simulink model "debut_de_qq"  (R2014a)
settings: Solver=ode45  StartTime=0.0  StopTime=10.0  RelTol=1e-3
undefined symbols (not defined in the file): K, KD, r, Ti
libraries: lib_robotRP x2
settings Model: Creator=2asri13  LastModifiedBy=2asri13

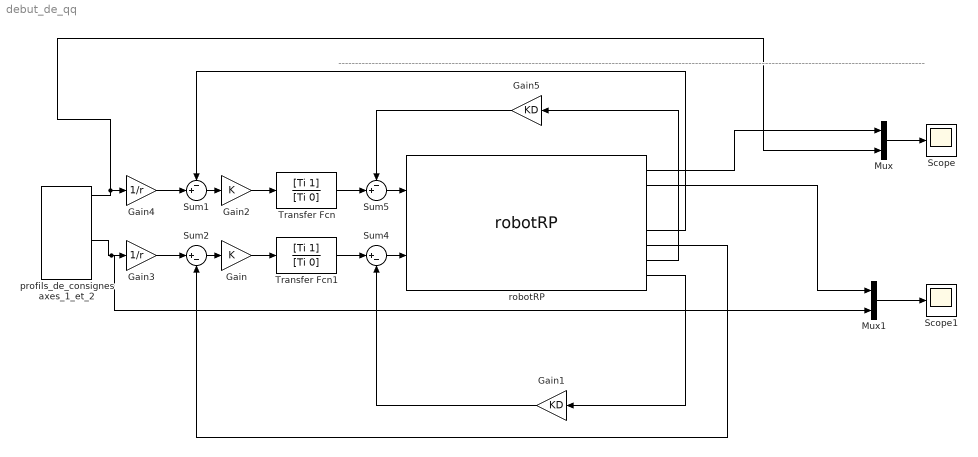
== system debut_de_qq ==
  note: --------------------------------------------------------------------------------------------------------------------------------------------------------------------------------
  Gain : Gain  Gain=K
  Gain1 : Gain  Gain=KD
  Gain2 : Gain  Gain=K
  Gain3 : Gain  Gain=1/r
  Gain4 : Gain  Gain=1/r
  Gain5 : Gain  Gain=KD
  Mux : Mux  Inputs=2
  Mux1 : Mux  Inputs=2
  Scope : Scope
  Scope1 : Scope
  Sum1 : Sum  Inputs=-+|
  Sum2 : Sum  Inputs=|+-
  Sum4 : Sum  Inputs=|+-
  Sum5 : Sum  Inputs=-+|
  Transfer Fcn : TransferFcn  Numerator=[Ti 1]  Denominator=[Ti 0]
  Transfer Fcn1 : TransferFcn  Numerator=[Ti 1]  Denominator=[Ti 0]
  profils_de_consignes axes_1_et_2 : lib_robotRP/profils_de_consignes axes_1_et_2
  robotRP : lib_robotRP/robotRP  vecteur_theta_dtheta_initial=[0 ; 0.5/r ; 0 ; 0]  m=15  gX=0  gY=0  F1=0  F2=0  H1=0  H2=0  Km_sur_R=0.3  Jm=0.01  Beff=0.0125  r=r
  wires:
  robotRP/1 -> Mux/1
  robotRP/2 -> Mux1/1
  robotRP/5 -> Sum1/1
  robotRP/6 -> Sum2/2
  robotRP/7 -> Gain5/1
  robotRP/8 -> Gain1/1
  Gain5/1 -> Sum5/1
  Gain1/1 -> Sum4/2
  Sum4/1 -> robotRP/2
  Sum5/1 -> robotRP/1
  Sum1/1 -> Gain2/1
  Sum2/1 -> Gain/1
  Gain4/1 -> Sum1/2
  Gain3/1 -> Sum2/1
  profils_de_consignes axes_1_et_2/1 -> Gain4/1, Mux/2
  profils_de_consignes axes_1_et_2/4 -> Mux1/2, Gain3/1
  Mux1/1 -> Scope1/1
  Mux/1 -> Scope/1
  Gain2/1 -> Transfer Fcn/1
  Transfer Fcn/1 -> Sum5/2
  Gain/1 -> Transfer Fcn1/1
  Transfer Fcn1/1 -> Sum4/1
